simulink model "FuzzyPID_Quadrotor"  (R2025a)
settings: Solver=ode8  StartTime=0.0  StopTime=40  FixedStep=0.002  RelTol=1e-3
undefined symbols (not defined in the file): b, d, g, Ir, Ixx, Iyy, Izz, k_phi, Ki, Kp, kx, l, m
libraries: fuzblock x6, slpidlib x6, simulink x2
(part 1 of 2)
settings Model: SimulationMode=accelerator  Creator=Viết Khoa  LastModifiedBy=Viết Khoa

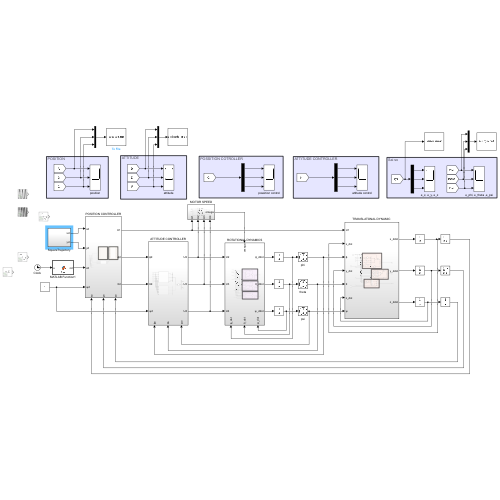
[thumbnail: Simulink's stored preview of the top-level diagram]
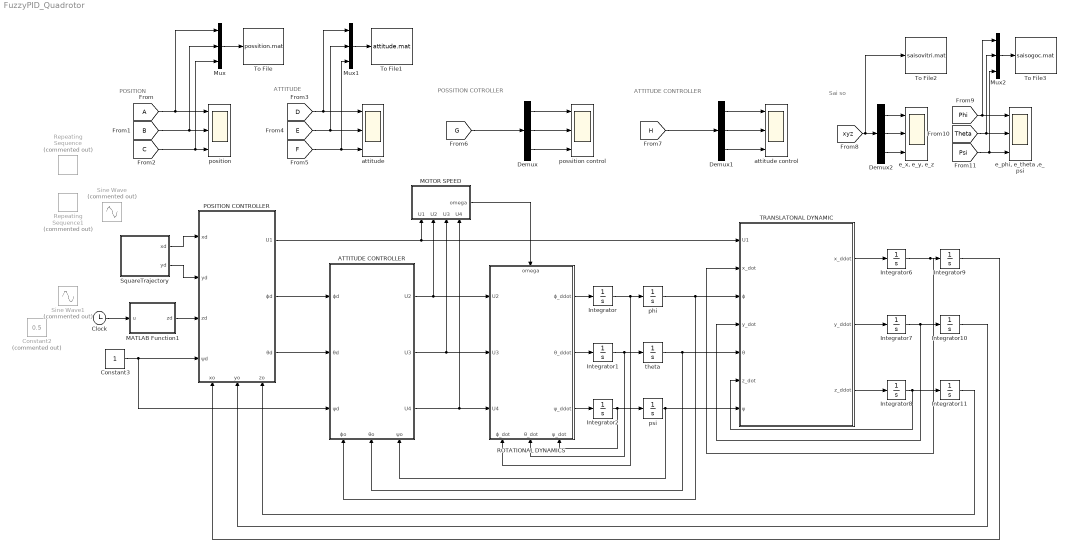
== system FuzzyPID_Quadrotor ==
  note: Sai so
  note: ATTITUDE CONTROLLER
  note: POSSITION COTROLLER
  note: ATTITUDE
  note: POSITION
  ATTITUDE CONTROLLER : Subsystem
      settings: PortSchema="{\"entries\":[{\"content\":{\"sides\":[{\"content\":{\"connectorIds\":[\"In1\",\"In2\",\"In3\"]},\"type\":\"ConnectorPlacement.EquallySpacedRectSide\",\"uuid\":\"4bf47d75-1d65-400d-a9d7-dbab3bfa16fd\"},{\"content\":{\"connectorIds\":[\"Out1\",\"Out2\",\"Out3\"],\"side\":\"RIGHT\"},\"type\":\"ConnectorPlacement.EquallySpacedRectSide\",\"uuid\":\"3ee65417-4730-4e86-9f3b-108f9b220256\"},{\"content\":{\"side\":\"TOP\"},\"type\":\"ConnectorPlacement.EquallySpacedRectSide\",\"uuid\":\"7506844b-c41f-4bd0-8d08-56ad7b5c83a6\"},{\"content\":{\"connectorIds\":[\"In4\",\"In5\",\"In6\"],\"side\":\"BOTTOM\"},\"type\":\"ConnectorPlacement.EquallySpacedRectSide\",\"uuid\":\"6a86c302-75aa-4327-998b-e6dc54af4631\"}]},\"type\":\"ConnectorPlacement.EquallySpacedConnector\",\"uuid\":\"8a896813-9530-416f-9d14-fc8134ed92a5\"}],\"packageUris\":[\"http://schema.mathworks.com/mf0/Connector/R2020b\"],\"version\":\"1.0\"}"
  Clock : Clock
      settings: Decimation=5
  Constant2 : Constant  Commented=on  Value=0.5
  Constant3 : Constant
  Demux : Demux  Outputs=3
  Demux1 : Demux  Outputs=3
  Demux2 : Demux  Outputs=3
  From : From  TagVisibility=global
  Integrator{,1..2,6..8,11} (7 alike) : Integrator
  Integrator10 : Integrator  LimitOutput=on  UpperSaturationLimit=100  LowerSaturationLimit=-100
  Integrator9 : Integrator  LimitOutput=on  UpperSaturationLimit=100  LowerSaturationLimit=-100
  MATLAB Function1 : MATLAB Function  TreatAsAtomicUnit=on
  MOTOR SPEED : Subsystem
      settings: PortSchema="{\"entries\":[{\"content\":{\"sides\":[{\"content\":{},\"type\":\"ConnectorPlacement.EquallySpacedRectSide\",\"uuid\":\"ed6e6d8d-e7bc-483a-ade7-47978a21bcb7\"},{\"content\":{\"connectorIds\":[\"Out1\"],\"side\":\"RIGHT\"},\"type\":\"ConnectorPlacement.EquallySpacedRectSide\",\"uuid\":\"acdfb20e-7f8e-459d-9194-6fd83a2c6b9b\"},{\"content\":{\"side\":\"TOP\"},\"type\":\"ConnectorPlacement.EquallySpacedRectSide\",\"uuid\":\"108cd3b7-cbe9-442f-8db2-72975fa6e768\"},{\"content\":{\"connectorIds\":[\"In1\",\"In2\",\"In3\",\"In4\"],\"side\":\"BOTTOM\"},\"type\":\"ConnectorPlacement.EquallySpacedRectSide\",\"uuid\":\"f7e31c23-3afe-47be-8aad-c67f1ef0a18a\"}]},\"type\":\"ConnectorPlacement.EquallySpacedConnector\",\"uuid\":\"b50d042a-fda9-4edf-aa4f-f774072a8c4f\"}],\"packageUris\":[\"http://schema.mathworks.com/mf0/Connector/R2020b\"],\"version\":\"1.0\"}"
  Mux : Mux  Inputs=3
  Mux1 : Mux  Inputs=3
  Mux2 : Mux  Inputs=3
  POSITION CONTROLLER : Subsystem
      settings: PortSchema="{\"entries\":[{\"content\":{\"sides\":[{\"content\":{\"connectorIds\":[\"In1\",\"In2\",\"In3\",\"In4\"]},\"type\":\"ConnectorPlacement.EquallySpacedRectSide\",\"uuid\":\"eaff3012-b374-4ff4-8d4a-29bbaff74213\"},{\"content\":{\"connectorIds\":[\"Out1\",\"Out2\",\"Out3\"],\"side\":\"RIGHT\"},\"type\":\"ConnectorPlacement.EquallySpacedRectSide\",\"uuid\":\"8b751115-4641-4ab1-9b2f-89aa7d40407f\"},{\"content\":{\"side\":\"TOP\"},\"type\":\"ConnectorPlacement.EquallySpacedRectSide\",\"uuid\":\"251f519b-9a79-4722-afff-0c5686202dfb\"},{\"content\":{\"connectorIds\":[\"In5\",\"In6\",\"In7\"],\"side\":\"BOTTOM\"},\"type\":\"ConnectorPlacement.EquallySpacedRectSide\",\"uuid\":\"18ce31f3-7bc4-45f8-83b4-9be4d1bc6b59\"}]},\"type\":\"ConnectorPlacement.EquallySpacedConnector\",\"uuid\":\"739509a0-8fec-462a-89d1-8b6a9a4571ac\"}],\"packageUris\":[\"http://schema.mathworks.com/mf0/Connector/R2020b\"],\"version\":\"1.0\"}"
  ROTATIONAL DYNAMICS : Subsystem
      settings: PortSchema="{\"entries\":[{\"content\":{\"sides\":[{\"content\":{\"connectorIds\":[\"In1\",\"In2\",\"In3\"]},\"type\":\"ConnectorPlacement.EquallySpacedRectSide\",\"uuid\":\"7bcebf77-1756-4e12-96a0-14289ff92643\"},{\"content\":{\"connectorIds\":[\"Out1\",\"Out2\",\"Out3\"],\"side\":\"RIGHT\"},\"type\":\"ConnectorPlacement.EquallySpacedRectSide\",\"uuid\":\"ba5ef720-59d3-4ec6-96cc-ef21a82cc408\"},{\"content\":{\"connectorIds\":[\"In4\"],\"side\":\"TOP\"},\"type\":\"ConnectorPlacement.EquallySpacedRectSide\",\"uuid\":\"de80adae-98be-49c2-8fe3-5182cf710150\"},{\"content\":{\"connectorIds\":[\"In5\",\"In6\",\"In7\"],\"side\":\"BOTTOM\"},\"type\":\"ConnectorPlacement.EquallySpacedRectSide\",\"uuid\":\"f6125003-ce59-4f76-bda5-387ee1b71a2b\"}]},\"type\":\"ConnectorPlacement.EquallySpacedConnector\",\"uuid\":\"a024e3ba-32fb-4ba4-b454-db7adc7fb913\"}],\"packageUris\":[\"http://schema.mathworks.com/mf0/Connector/R2020b\"],\"version\":\"1.0\"}"
  Repeating Sequence : simulink/Sources/Repeating Sequence  Commented=on  rep_seq_t=[0 2 4 6 8 10]  rep_seq_y=[0 0 2 2 0 0 ]
  Repeating Sequence1 : simulink/Sources/Repeating Sequence  Commented=on  rep_seq_t=[0 2 4 6 8 10]  rep_seq_y=[0 2 2 0 0 2 ]
  Sine Wave : Sin  Commented=on  Amplitude=2  Frequency=pi/10  SampleTime=0
  Sine Wave1 : Sin  Commented=on  Amplitude=2  Frequency=pi/10  Phase=pi/2  SampleTime=0
  SquareTrajectory : Subsystem
  "TRANSLATONAL DYNAMIC " : Subsystem
  To File : ToFile  Filename=possition.mat
  To File1 : ToFile  Filename=attitude.mat  SaveFormat=Timeseries
  To File2 : ToFile  Filename=saisovitri.mat
  To File3 : ToFile  Filename=saisogoc.mat
  attitude : Scope  NumInputPorts=3
      settings: ActiveDisplayYMinimum=-0.31829898344644053  ActiveDisplayYMaximum=0.3123395018117221
  attitude control : Scope  NumInputPorts=3
      settings: ActiveDisplayString=3  ActiveDisplayYMinimum=-26.113832641242233  ActiveDisplayYMaximum=59.012648071249139  DataLoggingVariableName=ScopeData3
  "e_phi, e_theta ,e_psi" : Scope  NumInputPorts=3
      settings: ActiveDisplayString=3  ActiveDisplayYMinimum=-0.23701033608813543  ActiveDisplayYMaximum=1.1374455928986817  YLabel=epsi  DataLoggingVariableName=ScopeData5
  "e_x, e_y, e_z" : Scope  NumInputPorts=3
      settings: ActiveDisplayString=3  ActiveDisplayYMinimum=-1.3848015109481584  ActiveDisplayYMaximum=6.8205335012164623  YLabel=ez  DataLoggingVariableName=ScopeData4
  phi : Integrator  WrapState=on
  position : Scope  NumInputPorts=3
      settings: ActiveDisplayYMinimum=-1.3944694562558515  ActiveDisplayYMaximum=12.140863842930267
  possition control : Scope  NumInputPorts=3
      settings: ActiveDisplayString=3  ActiveDisplayYMinimum=-3.1076811932529651  ActiveDisplayYMaximum=19.789742354805885  YLabel=Uz  DataLoggingVariableName=ScopeData2
  psi : Integrator  WrapState=on
  theta : Integrator  WrapState=on
  wires:
  Constant3/1 -> ATTITUDE CONTROLLER/3(ψd), POSITION CONTROLLER/4(ψd)
  POSITION CONTROLLER/2(ϕd) -> ATTITUDE CONTROLLER/1(ϕd)
  POSITION CONTROLLER/3(θd) -> ATTITUDE CONTROLLER/2(θd)
  ATTITUDE CONTROLLER/3(U4) -> ROTATIONAL DYNAMICS/3(U4), MOTOR SPEED/4(U4)
  ATTITUDE CONTROLLER/2(U3) -> MOTOR SPEED/3(U3), ROTATIONAL DYNAMICS/2(U3)
  ATTITUDE CONTROLLER/1(U2) -> ROTATIONAL DYNAMICS/1(U2), MOTOR SPEED/2(U2)
  MOTOR SPEED/1(omega) -> ROTATIONAL DYNAMICS/4(omega)
  ROTATIONAL DYNAMICS/1(ϕ_ddot) -> Integrator/1
  Integrator/1 -> ROTATIONAL DYNAMICS/5(ϕ_dot), phi/1
  ROTATIONAL DYNAMICS/2(θ_ddot) -> Integrator1/1
  Integrator1/1 -> ROTATIONAL DYNAMICS/6(θ_dot), theta/1
  ROTATIONAL DYNAMICS/3(ψ_ddot) -> Integrator2/1
  phi/1 -> ATTITUDE CONTROLLER/4(ϕo), "TRANSLATONAL DYNAMIC "/3(ϕ)
  theta/1 -> "TRANSLATONAL DYNAMIC "/5(θ), ATTITUDE CONTROLLER/5(θo)
  psi/1 -> ATTITUDE CONTROLLER/6(ψo), "TRANSLATONAL DYNAMIC "/7(ψ)
  Integrator2/1 -> ROTATIONAL DYNAMICS/7(ψ_dot), psi/1
  POSITION CONTROLLER/1(U1) -> MOTOR SPEED/1(U1), "TRANSLATONAL DYNAMIC "/1(U1)
  "TRANSLATONAL DYNAMIC "/1(x_ddot) -> Integrator6/1
  Integrator6/1 -> "TRANSLATONAL DYNAMIC "/2(x_dot), Integrator9/1
  "TRANSLATONAL DYNAMIC "/2(y_ddot) -> Integrator7/1
  Integrator7/1 -> "TRANSLATONAL DYNAMIC "/4(y_dot), Integrator10/1
  "TRANSLATONAL DYNAMIC "/3(z_ddot) -> Integrator8/1
  Integrator8/1 -> Integrator11/1, "TRANSLATONAL DYNAMIC "/6(z_dot)
  Integrator9/1 -> POSITION CONTROLLER/5(xo)
  Integrator10/1 -> POSITION CONTROLLER/6(yo)
  Integrator11/1 -> POSITION CONTROLLER/7(zo)
  [C] -> Mux/3, position/3
  [B] -> Mux/2, position/2
  From/1 -> Mux/1, position/1
  [D] -> Mux1/1, attitude/1
  [F] -> Mux1/3, attitude/3
  [E] -> Mux1/2, attitude/2
  [G] -> Demux/1
  Demux/1 -> possition control/1
  Demux/2 -> possition control/2
  Demux/3 -> possition control/3
  Demux1/3 -> attitude control/3
  Demux1/2 -> attitude control/2
  Demux1/1 -> attitude control/1
  [H] -> Demux1/1
  [Phi] -> Mux2/1, "e_phi, e_theta ,e_psi"/1
  [Theta] -> Mux2/2, "e_phi, e_theta ,e_psi"/2
  [Psi] -> Mux2/3, "e_phi, e_theta ,e_psi"/3
  [xyz] -> To File2/1, Demux2/1
  Demux2/1 -> "e_x, e_y, e_z"/1
  Demux2/2 -> "e_x, e_y, e_z"/2
  Demux2/3 -> "e_x, e_y, e_z"/3
  Clock/1 -> MATLAB Function1/1(u)
  MATLAB Function1/1(zd) -> POSITION CONTROLLER/3(zd)
  SquareTrajectory/1(xd) -> POSITION CONTROLLER/1(xd)
  SquareTrajectory/2(yd) -> POSITION CONTROLLER/2(yd)
  Mux/1 -> To File/1
  Mux1/1 -> To File1/1
  Mux2/1 -> To File3/1

== system FuzzyPID_Quadrotor/ATTITUDE CONTROLLER ==
  ϕd : Inport
  θd : Inport  Port=2
  ψd : Inport  Port=3
  ϕo : Inport  Port=4
  θo : Inport  Port=5
  ψo : Inport  Port=6
  Demux : Demux  Outputs=3
  FuzzyPID_Attitude : Subsystem
  Manual Switch : ManualSwitch
  Mux : Mux  Inputs=3
  Mux1 : Mux  Commented=on  Inputs=3
  Subsystem : Subsystem  Commented=on
  U2 : Outport
  U3 : Outport  Port=2
  U4 : Outport  Port=3
  wires:
  ϕd/1 -> Subsystem/1(ϕd), FuzzyPID_Attitude/1(ϕd)
  ϕo/1 -> Subsystem/2(ϕo), FuzzyPID_Attitude/2(ϕo)
  θd/1 -> Subsystem/3(θd), FuzzyPID_Attitude/3(θd)
  θo/1 -> Subsystem/4(θo), FuzzyPID_Attitude/4(θo)
  ψd/1 -> Subsystem/5(ψd), FuzzyPID_Attitude/5(ψd)
  ψo/1 -> Subsystem/6(ψo), FuzzyPID_Attitude/6(ψo)
  FuzzyPID_Attitude/2(U3) -> Mux/2
  FuzzyPID_Attitude/1(U2) -> Mux/1
  FuzzyPID_Attitude/3(U4) -> Mux/3
  Subsystem/2(U3) -> Mux1/2
  Subsystem/1(U2) -> Mux1/1
  Subsystem/3(U4) -> Mux1/3
  Mux/1 -> Manual Switch/1
  Mux1/1 -> Manual Switch/2
  Manual Switch/1 -> Demux/1
  Demux/3 -> U4/1
  Demux/2 -> U3/1
  Demux/1 -> U2/1

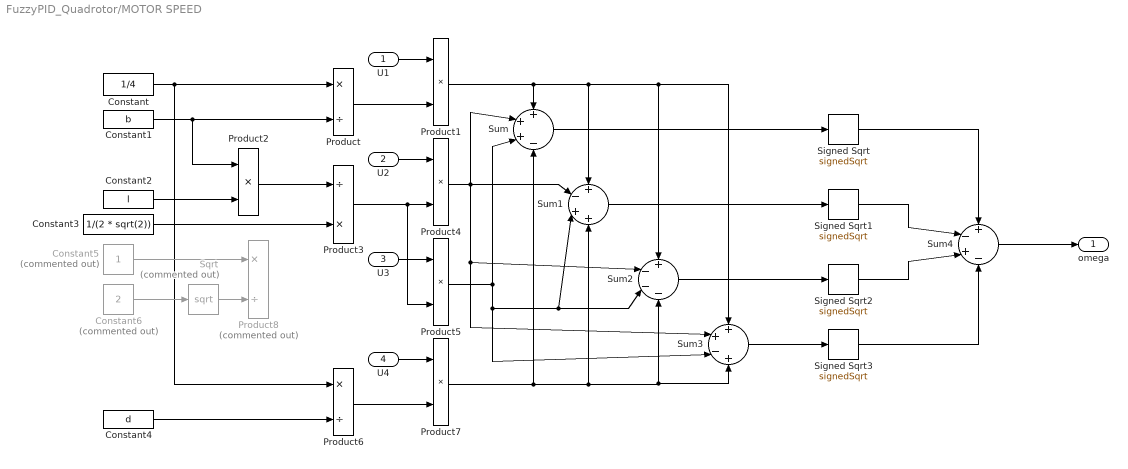
== system FuzzyPID_Quadrotor/MOTOR SPEED ==
  U1 : Inport
  U2 : Inport  Port=2
  U3 : Inport  Port=3
  U4 : Inport  Port=4
  Constant : Constant  Value=1/4
  Constant1 : Constant  Value=b
  Constant2 : Constant  Value=l
  Constant3 : Constant  Value=1/(2 * sqrt(2))
  Constant4 : Constant  Value=d
  Constant5 : Constant  Commented=on
  Constant6 : Constant  Commented=on  Value=2
  Product : Product  Inputs=*/
  Product{1..2,4..5,7} (5 alike) : Product
  Product3 : Product  Inputs=/*
  Product6 : Product  Inputs=*/
  Product8 : Product  Commented=on  Inputs=*/
  Signed Sqrt{,1..3} (4 alike) : Sqrt  Operator=signedSqrt
  Sqrt : Sqrt  Commented=on
  Sum : Sum  Inputs=+++-
  Sum1 : Sum  Inputs=+-++
  Sum2 : Sum  Inputs=+---
  Sum3 : Sum  Inputs=++-+
  Sum4 : Sum  Inputs=+-+-
  omega : Outport
  wires:
  Constant/1 -> Product6/1, Product/1
  Constant1/1 -> Product2/1, Product/2
  U1/1 -> Product1/1
  Product/1 -> Product1/2
  Constant2/1 -> Product2/2
  Product2/1 -> Product3/1
  U2/1 -> Product4/1
  Product3/1 -> Product5/2, Product4/2
  U3/1 -> Product5/1
  Constant4/1 -> Product6/2
  Product6/1 -> Product7/2
  U4/1 -> Product7/1
  Product1/1 -> Sum/1, Sum2/1, Sum3/1, Sum1/1
  Product4/1 -> Sum2/2, Sum3/2, Sum/2, Sum1/2
  Product5/1 -> Sum3/3, Sum1/3, Sum2/3, Sum/3
  Product7/1 -> Sum/4, Sum3/4, Sum2/4, Sum1/4
  Sum/1 -> Signed Sqrt/1
  Sum1/1 -> Signed Sqrt1/1
  Sum2/1 -> Signed Sqrt2/1
  Sum3/1 -> Signed Sqrt3/1
  Signed Sqrt/1 -> Sum4/1
  Signed Sqrt1/1 -> Sum4/2
  Signed Sqrt2/1 -> Sum4/3
  Signed Sqrt3/1 -> Sum4/4
  Sum4/1 -> omega/1
  Constant6/1 -> Sqrt/1
  Sqrt/1 -> Product8/2
  Constant5/1 -> Product8/1
  Constant3/1 -> Product3/2

== system FuzzyPID_Quadrotor/POSITION CONTROLLER ==
  note: CACULATION DESIRED ROLL AND PITCH, THUST
  note: BỘ ĐIỀU KHIỂN VỊ TRÍ
  xd : Inport
  yd : Inport  Port=2
  zd : Inport  Port=3
  ψd : Inport  Port=4
  xo : Inport  Port=5
  yo : Inport  Port=6
  zo : Inport  Port=7
  Demux : Demux  Commented=on  Outputs=6
  Demux1 : Demux  Outputs=6
  FUZZY PID POSITION : Subsystem  Commented=on
  Goto : Goto  TagVisibility=global
  Mux : Mux  Inputs=6
  Mux1 : Mux  Inputs=2
  Mux2 : Mux  Inputs=2
  Mux3 : Mux  Inputs=2
  Subsystem : Subsystem
      settings: PortSchema="{\"entries\":[{\"content\":{\"sides\":[{\"content\":{\"connectorIds\":[\"In1\",\"In2\",\"In3\"]},\"type\":\"ConnectorPlacement.EquallySpacedRectSide\",\"uuid\":\"734b09d6-8ba9-424b-aad8-7b68aeaa8799\"},{\"content\":{\"connectorIds\":[\"Out1\",\"Out2\",\"Out3\"],\"side\":\"RIGHT\"},\"type\":\"ConnectorPlacement.EquallySpacedRectSide\",\"uuid\":\"ae7a8814-eaf7-43aa-9eb5-210d717eae53\"},{\"content\":{\"side\":\"TOP\"},\"type\":\"ConnectorPlacement.EquallySpacedRectSide\",\"uuid\":\"c79c257a-0698-4fb1-979a-f95adc922051\"},{\"content\":{\"connectorIds\":[\"In4\"],\"side\":\"BOTTOM\"},\"type\":\"ConnectorPlacement.EquallySpacedRectSide\",\"uuid\":\"97cb2459-45e5-4eb8-bf6c-59a8c59ceda8\"}]},\"type\":\"ConnectorPlacement.EquallySpacedConnector\",\"uuid\":\"b23e5638-8d2f-4e41-ba88-ebe95de464d7\"}],\"packageUris\":[\"http://schema.mathworks.com/mf0/Connector/R2020b\"],\"version\":\"1.0\"}"
  Subsystem2 : Subsystem
  U1 : Outport
  ϕd : Outport  Port=2
  θd : Outport  Port=3
  tag scope: B=global, C=global
  wires:
  ψd/1 -> Subsystem/4(ψd)
  Subsystem/1(U1) -> U1/1
  Subsystem/2(ϕd) -> ϕd/1
  Subsystem/3(θd) -> θd/1
  xd/1 -> Mux/1, Mux1/1
  yd/1 -> Mux2/1, Mux/2
  zd/1 -> Mux3/1, Mux/3
  xo/1 -> Mux/4, Mux1/2
  yo/1 -> Mux2/2, Mux/5
  zo/1 -> Mux3/2, Mux/6
  Demux/6 -> FUZZY PID POSITION/6(zo)
  Demux/5 -> FUZZY PID POSITION/5(yo)
  Demux/4 -> FUZZY PID POSITION/4(xo)
  Demux/3 -> FUZZY PID POSITION/3(zd)
  Demux/2 -> FUZZY PID POSITION/2(yd)
  Demux/1 -> FUZZY PID POSITION/1(xd)
  Mux/1 -> Demux/1, Demux1/1
  Demux1/1 -> Subsystem2/1(xd)
  Demux1/2 -> Subsystem2/2(yd)
  Demux1/3 -> Subsystem2/3(zd)
  Demux1/4 -> Subsystem2/4(xo)
  Demux1/5 -> Subsystem2/5(yo)
  Demux1/6 -> Subsystem2/6(zo)
  Mux1/1 -> Goto/1
  Mux2/1 -> [B]
  Mux3/1 -> [C]
  Subsystem2/1(Ux) -> Subsystem/1(Ux)
  Subsystem2/2(Uy) -> Subsystem/2(Uy)
  Subsystem2/3(Uz) -> Subsystem/3(Uz)

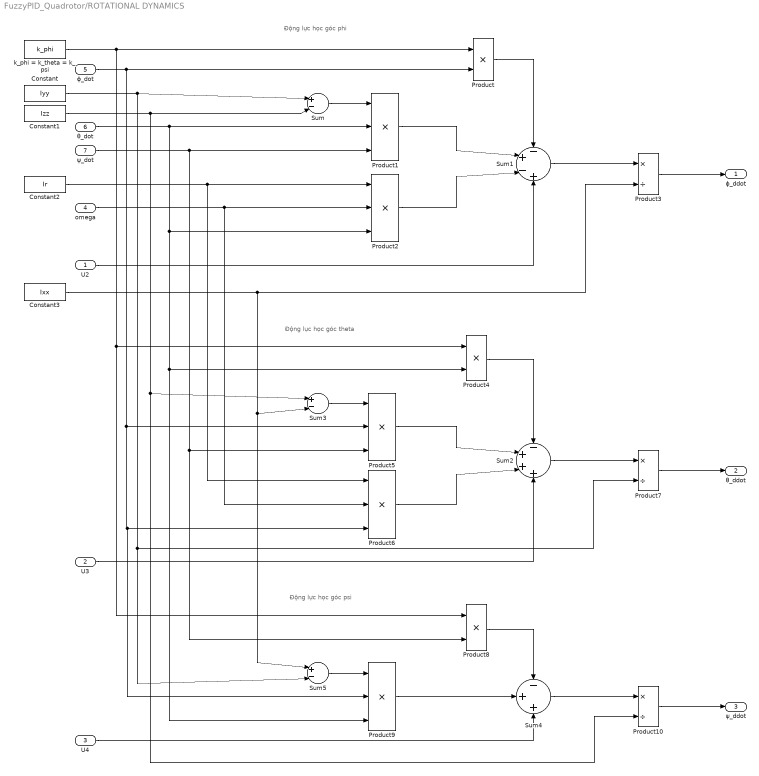
== system FuzzyPID_Quadrotor/ROTATIONAL DYNAMICS ==
  note: Động lực học góc psi
  note: Động lục học góc theta
  note: Động lực học góc phi
  U2 : Inport
  U3 : Inport  Port=2
  U4 : Inport  Port=3
  omega : Inport  Port=4
  ϕ_dot : Inport  Port=5
  θ_dot : Inport  Port=6
  ψ_dot : Inport  Port=7
  Constant : Constant  Value=Iyy
  Constant1 : Constant  Value=Izz
  Constant2 : Constant  Value=Ir
  Constant3 : Constant  Value=Ixx
  Product : Product
  Product{1..2,5..6,9} (5 alike) : Product  Inputs=3
  Product10 : Product  Inputs=*/
  Product3 : Product  Inputs=*/
  Product4 : Product
  Product7 : Product  Inputs=*/
  Product8 : Product
  Sum : Sum  Inputs=|+-|
  Sum1 : Sum  Inputs=-+-+
  Sum2 : Sum  Inputs=-+++
  Sum3 : Sum  Inputs=|+-|
  Sum4 : Sum  Inputs=-++
  Sum5 : Sum  Inputs=|+-|
  k_phi = k_theta = k_psi : Constant  Value=k_phi
  ϕ_ddot : Outport
  θ_ddot : Outport  Port=2
  ψ_ddot : Outport  Port=3
  wires:
  k_phi = k_theta = k_psi/1 -> Product8/1, Product4/1, Product/1
  ϕ_dot/1 -> Product/2, Product5/2, Product9/2, Product6/3
  Constant/1 -> Product7/2, Sum5/2, Sum/1
  Constant1/1 -> Sum3/1, Product10/2, Sum/2
  Sum/1 -> Product1/1
  Product/1 -> Sum1/1
  Product1/1 -> Sum1/2
  Constant2/1 -> Product6/1, Product2/1
  omega/1 -> Product6/2, Product2/2
  Product2/1 -> Sum1/3
  U2/1 -> Sum1/4
  Sum1/1 -> Product3/1
  Constant3/1 -> Sum3/2, Sum5/1, Product3/2
  Product3/1 -> ϕ_ddot/1
  θ_dot/1 -> Product4/2, Product9/3, Product2/3, Product1/2
  Product4/1 -> Sum2/1
  Sum3/1 -> Product5/1
  Product5/1 -> Sum2/2
  Product6/1 -> Sum2/3
  Sum2/1 -> Product7/1
  Product7/1 -> θ_ddot/1
  ψ_dot/1 -> Product8/2, Product5/3, Product1/3
  Product8/1 -> Sum4/1
  Sum5/1 -> Product9/1
  Product9/1 -> Sum4/2
  U3/1 -> Sum2/4
  U4/1 -> Sum4/3
  Sum4/1 -> Product10/1
  Product10/1 -> ψ_ddot/1

== system FuzzyPID_Quadrotor/SquareTrajectory ==
  Clock : Clock
      settings: Decimation=5
  Clock1 : Clock
      settings: Decimation=5
  MATLAB Function : MATLAB Function  TreatAsAtomicUnit=on
  MATLAB Function1 : MATLAB Function  TreatAsAtomicUnit=on
  To Workspace : ToWorkspace  VariableName=Time  SampleTime=-1
  To Workspace1 : ToWorkspace  VariableName=xd  SampleTime=-1
  To Workspace2 : ToWorkspace  VariableName=yd  SampleTime=-1
  xd : Outport
  yd : Outport  Port=2
  wires:
  Clock/1 -> MATLAB Function1/1(u), MATLAB Function/1(u)
  Clock1/1 -> To Workspace/1
  MATLAB Function1/1(xd) -> To Workspace1/1, xd/1
  MATLAB Function/1(yd) -> To Workspace2/1, yd/1

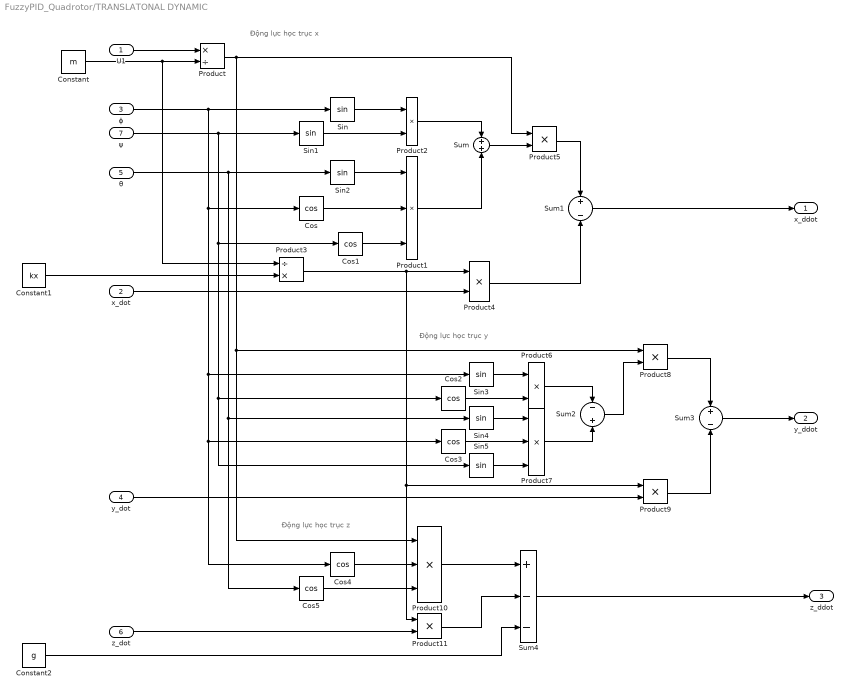
== system FuzzyPID_Quadrotor/TRANSLATONAL DYNAMIC  ==
  note: Động lực học trục z
  note: Động lực học trục y
  note: Động lực học trục x
  U1 : Inport
  x_dot : Inport  Port=2
  ϕ : Inport  Port=3
  y_dot : Inport  Port=4
  θ : Inport  Port=5
  z_dot : Inport  Port=6
  ψ : Inport  Port=7
  Constant : Constant  Value=m
  Constant1 : Constant  Value=kx
  Constant2 : Constant  Value=g
  Cos{,1..5} (6 alike) : Trigonometry  Operator=cos
  Product : Product  Inputs=*/
  Product1 : Product  Inputs=3
  Product10 : Product  Inputs=3
  Product{2,4..6,8..9,11} (7 alike) : Product
  Product3 : Product  Inputs=/*
  Product7 : Product  Inputs=3
  Sin{,1..5} (6 alike) : Trigonometry
  Sum : Sum  Inputs=+|+
  Sum1 : Sum  Inputs=+|-
  Sum2 : Sum  Inputs=-|+
  Sum3 : Sum  Inputs=+|-
  Sum4 : Sum  Inputs=+--
  x_ddot : Outport
  y_ddot : Outport  Port=2
  z_ddot : Outport  Port=3
  wires:
  U1/1 -> Product/1
  Constant/1 -> Product/2, Product3/1
  ϕ/1 -> Sin/1, Cos/1, Sin3/1, Cos4/1, Cos3/1
  Sin/1 -> Product2/1
  ψ/1 -> Sin1/1, Cos1/1, Cos2/1, Sin5/1
  Sin1/1 -> Product2/2
  θ/1 -> Sin4/1, Cos5/1, Sin2/1
  Sin2/1 -> Product1/1
  Cos/1 -> Product1/2
  Cos1/1 -> Product1/3
  Product2/1 -> Sum/1
  Product1/1 -> Sum/2
  Constant1/1 -> Product3/2
  Product3/1 -> Product11/1, Product9/1, Product4/1
  x_dot/1 -> Product4/2
  Product4/1 -> Sum1/2
  Sum/1 -> Product5/2
  Product5/1 -> Sum1/1
  Sin3/1 -> Product6/1
  Cos2/1 -> Product6/2
  Sin4/1 -> Product7/1
  Cos3/1 -> Product7/2
  Sin5/1 -> Product7/3
  Product6/1 -> Sum2/1
  Product7/1 -> Sum2/2
  Sum2/1 -> Product8/2
  y_dot/1 -> Product9/2
  Product8/1 -> Sum3/1
  Product9/1 -> Sum3/2
  Product/1 -> Product8/1, Product10/1, Product5/1
  Cos4/1 -> Product10/2
  Cos5/1 -> Product10/3
  z_dot/1 -> Product11/2
  Product10/1 -> Sum4/1
  Product11/1 -> Sum4/2
  Constant2/1 -> Sum4/3
  Sum1/1 -> x_ddot/1
  Sum3/1 -> y_ddot/1
  Sum4/1 -> z_ddot/1

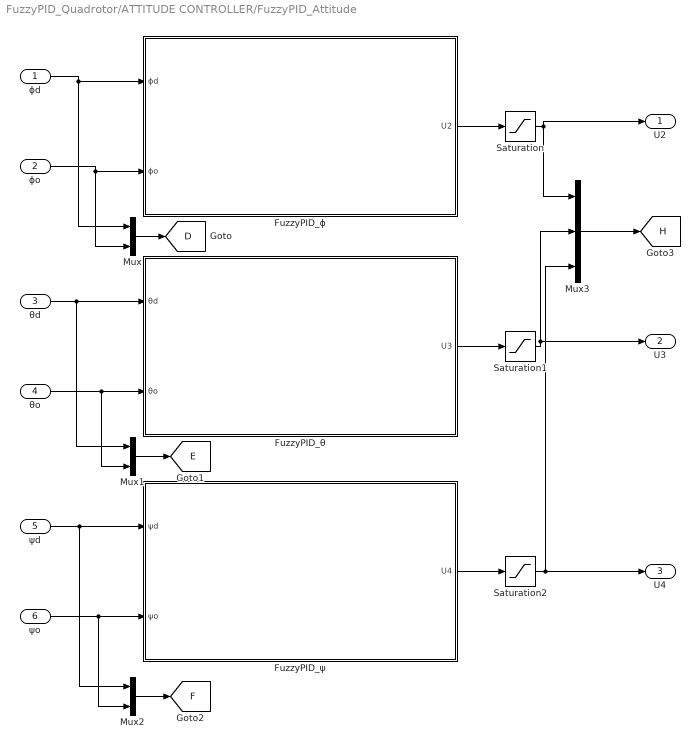
== system FuzzyPID_Quadrotor/ATTITUDE CONTROLLER/FuzzyPID_Attitude ==
  ϕd : Inport
  ϕo : Inport  Port=2
  θd : Inport  Port=3
  θo : Inport  Port=4
  ψd : Inport  Port=5
  ψo : Inport  Port=6
  FuzzyPID_θ : Subsystem
  FuzzyPID_ψ : Subsystem
  FuzzyPID_ϕ : Subsystem
  Mux : Mux  Inputs=2
  Mux1 : Mux  Inputs=2
  Mux2 : Mux  Inputs=2
  Mux3 : Mux  Inputs=3
  Saturation : Saturate  UpperLimit=500  LowerLimit=-500
  Saturation1 : Saturate  UpperLimit=500  LowerLimit=-500
  Saturation2 : Saturate  UpperLimit=500  LowerLimit=-500
  U2 : Outport
  U3 : Outport  Port=2
  U4 : Outport  Port=3
  tag scope: D=global, E=global, F=global, H=global
  wires:
  ϕd/1 -> Mux/1, FuzzyPID_ϕ/1(ϕd)
  ψd/1 -> Mux2/1, FuzzyPID_ψ/1(ψd)
  Saturation1/1 -> U3/1, Mux3/2
  ψo/1 -> Mux2/2, FuzzyPID_ψ/2(ψo)
  Mux2/1 -> [F]
  ϕo/1 -> Mux/2, FuzzyPID_ϕ/2(ϕo)
  Saturation/1 -> U2/1, Mux3/1
  θo/1 -> Mux1/2, FuzzyPID_θ/2(θo)
  FuzzyPID_ψ/1(U4) -> Saturation2/1
  Saturation2/1 -> U4/1, Mux3/3
  Mux/1 -> [D]
  θd/1 -> Mux1/1, FuzzyPID_θ/1(θd)
  FuzzyPID_ϕ/1(U2) -> Saturation/1
  FuzzyPID_θ/1(U3) -> Saturation1/1
  Mux3/1 -> [H]
  Mux1/1 -> [E]

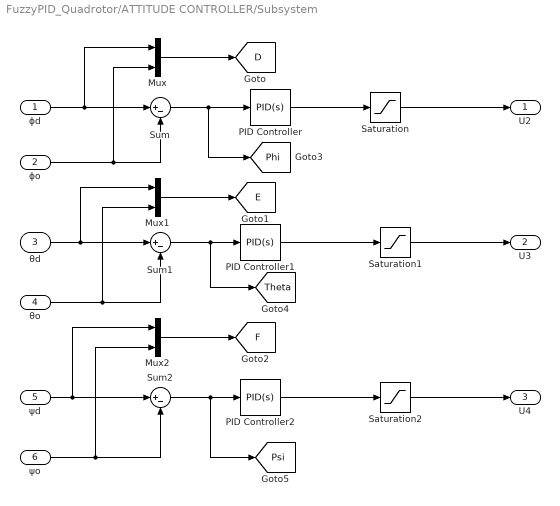
== system FuzzyPID_Quadrotor/ATTITUDE CONTROLLER/Subsystem ==
  ϕd : Inport
  ϕo : Inport  Port=2
  θd : Inport  Port=3
  θo : Inport  Port=4
  ψd : Inport  Port=5
  ψo : Inport  Port=6
  Mux : Mux  Inputs=2
  Mux1 : Mux  Inputs=2
  Mux2 : Mux  Inputs=2
  PID Controller : slpidlib/PID Controller  Controller=PID  Form=Parallel  TimeDomain=Continuous-time  UseExternalTs=off  SampleTime=-1  IntegratorMethod=Forward Euler  FilterMethod=Forward Euler  ControllerParametersSource=internal  P=1  I=0.01  UseKiTs=off  D=0.1  UseExternalDerivativeSource=off  N=0.0166910746973265  UseFilter=on  TunerSelectOption=Transfer Function Based (PID Tuner App)  InitialConditionSource=internal  InitialConditionForIntegrator=0  InitialConditionForFilter=0  DifferentiatorICPrevScaledInput=0  ExternalReset=none  TrackingMode=off  Kt=1  LimitOutput=off  SatLimitsSource=internal  UpperSaturationLimit=inf  LowerSaturationLimit=-inf  LinearizeAsGain=on  AntiWindupMode=none  Kb=1  LimitIntegrator=off  UpperIntegratorSaturationLimit=inf  LowerIntegratorSaturationLimit=-inf  POutMin=[]  POutMax=[]  IOutMin=[]  IOutMax=[]  DOutMin=[]  DOutMax=[]  NOutMin=[]  NOutMax=[]  SumOutMin=[]  SumOutMax=[]  SaturationOutMin=[]  SaturationOutMax=[]  PParamMin=[]  PParamMax=[]  IParamMin=[]  IParamMax=[]  DParamMin=[]  DParamMax=[]  NParamMin=[]  NParamMax=[]  KbParamMin=[]  KbParamMax=[]  KtParamMin=[]  KtParamMax=[]  KbOutMin=[]  KbOutMax=[]  KtOutMin=[]  KtOutMax=[]  IntegratorOutMin=[]  IntegratorOutMax=[]  FilterOutMin=[]  FilterOutMax=[]  SumI1OutMin=[]  SumI1OutMax=[]  SumI2OutMin=[]  SumI2OutMax=[]  SumI3OutMin=[]  SumI3OutMax=[]  SumI4OutMin=[]  SumI4OutMax=[]  SumDOutMin=[]  SumDOutMax=[]  DifferentiatorOutMin=[]  DifferentiatorOutMax=[]  FilterDiffOutCoefMin=[]  FilterDiffOutCoefMax=[]  ReciprocalOutMin=[]  ReciprocalOutMax=[]  SumDenOutMin=[]  SumDenOutMax=[]  SumNumOutMin=[]  SumNumOutMax=[]  DivideOutMin=[]  DivideOutMax=[]  UdiffTsProdOutMin=[]  UdiffTsProdOutMax=[]  NTsProdOutMin=[]  NTsProdOutMax=[]  UintegralTsProdOutMin=[]  UintegralTsProdOutMax=[]  UngainTsProdOutMin=[]  UngainTsProdOutMax=[]  ClampingZeroOutDataTypeStr=Inherit: Inherit via back propagation  ClampingZeroOutMin=[]  ClampingZeroOutMax=[]  FilterDenConstantOutDataTypeStr=Inherit: Inherit via back propagation  FilterDenConstantOutMin=[]  FilterDenConstantOutMax=[]  PCopyOutDataTypeStr=Inherit: Inherit via back propagation  PCopyOutMin=[]  PCopyOutMax=[]  NCopyOutDataTypeStr=Inherit: Inherit via back propagation  NCopyOutMin=[]  NCopyOutMax=[]  IntegratorContinuousStateAttributes=''  IntegratorStateMustResolveToSignalObject=off  IntegratorRTWStateStorageClass=Auto  FilterContinuousStateAttributes=''  FilterStateMustResolveToSignalObject=off  FilterRTWStateStorageClass=Auto  ParallelPVariant=InternalParameters  IdealPVariant=Disabled  IVariant=InternalParameters  DVariant=InternalParameters  IntegratorVariant=Continuous  SatVariant=Disabled  AWVariant=Passthrough  PCopyVariant=Disabled  TRVariant=Disabled  FdbkBlocksVariant=Forward  IdealPFdbkVariant=Disabled  SatFdbkVariant=Disabled  DerivativeFilterVariant=ContFilter  NVariant=InternalParameters  NCopyVariant=Disabled  FilterICVariant=InternalICsFilter  IntegratorICVariant=InternalICs  ExternalResetVariant=Disabled  TRSumVariant=Passthrough  SumFdbkVariant=Disabled  SumVariant=Sum_PID  TsampFilterVariant=InternalTs  TsampNgainVariant=Passthrough  TsampIntegralVariant=Disabled_SignalSpec  ExternalSaturationOutDataTypeStr=Inherit: Same as second input  DerivativeSourceVariant=ErrorSignal  PreIntVariant=InternalPreInt
  PID Controller1 : slpidlib/PID Controller  Controller=PID  Form=Parallel  TimeDomain=Continuous-time  UseExternalTs=off  SampleTime=-1  IntegratorMethod=Forward Euler  FilterMethod=Forward Euler  ControllerParametersSource=internal  P=1  I=0.01  UseKiTs=off  D=0.1  UseExternalDerivativeSource=off  N=100  UseFilter=on  TunerSelectOption=Transfer Function Based (PID Tuner App)  InitialConditionSource=internal  InitialConditionForIntegrator=0  InitialConditionForFilter=0  DifferentiatorICPrevScaledInput=0  ExternalReset=none  TrackingMode=off  Kt=1  LimitOutput=off  SatLimitsSource=internal  UpperSaturationLimit=inf  LowerSaturationLimit=-inf  LinearizeAsGain=on  AntiWindupMode=none  Kb=1  LimitIntegrator=off  UpperIntegratorSaturationLimit=inf  LowerIntegratorSaturationLimit=-inf  POutMin=[]  POutMax=[]  IOutMin=[]  IOutMax=[]  DOutMin=[]  DOutMax=[]  NOutMin=[]  NOutMax=[]  SumOutMin=[]  SumOutMax=[]  SaturationOutMin=[]  SaturationOutMax=[]  PParamMin=[]  PParamMax=[]  IParamMin=[]  IParamMax=[]  DParamMin=[]  DParamMax=[]  NParamMin=[]  NParamMax=[]  KbParamMin=[]  KbParamMax=[]  KtParamMin=[]  KtParamMax=[]  KbOutMin=[]  KbOutMax=[]  KtOutMin=[]  KtOutMax=[]  IntegratorOutMin=[]  IntegratorOutMax=[]  FilterOutMin=[]  FilterOutMax=[]  SumI1OutMin=[]  SumI1OutMax=[]  SumI2OutMin=[]  SumI2OutMax=[]  SumI3OutMin=[]  SumI3OutMax=[]  SumI4OutMin=[]  SumI4OutMax=[]  SumDOutMin=[]  SumDOutMax=[]  DifferentiatorOutMin=[]  DifferentiatorOutMax=[]  FilterDiffOutCoefMin=[]  FilterDiffOutCoefMax=[]  ReciprocalOutMin=[]  ReciprocalOutMax=[]  SumDenOutMin=[]  SumDenOutMax=[]  SumNumOutMin=[]  SumNumOutMax=[]  DivideOutMin=[]  DivideOutMax=[]  UdiffTsProdOutMin=[]  UdiffTsProdOutMax=[]  NTsProdOutMin=[]  NTsProdOutMax=[]  UintegralTsProdOutMin=[]  UintegralTsProdOutMax=[]  UngainTsProdOutMin=[]  UngainTsProdOutMax=[]  ClampingZeroOutDataTypeStr=Inherit: Inherit via back propagation  ClampingZeroOutMin=[]  ClampingZeroOutMax=[]  FilterDenConstantOutDataTypeStr=Inherit: Inherit via back propagation  FilterDenConstantOutMin=[]  FilterDenConstantOutMax=[]  PCopyOutDataTypeStr=Inherit: Inherit via back propagation  PCopyOutMin=[]  PCopyOutMax=[]  NCopyOutDataTypeStr=Inherit: Inherit via back propagation  NCopyOutMin=[]  NCopyOutMax=[]  IntegratorContinuousStateAttributes=''  IntegratorStateMustResolveToSignalObject=off  IntegratorRTWStateStorageClass=Auto  FilterContinuousStateAttributes=''  FilterStateMustResolveToSignalObject=off  FilterRTWStateStorageClass=Auto  ParallelPVariant=InternalParameters  IdealPVariant=Disabled  IVariant=InternalParameters  DVariant=InternalParameters  IntegratorVariant=Continuous  SatVariant=Disabled  AWVariant=Passthrough  PCopyVariant=Disabled  TRVariant=Disabled  FdbkBlocksVariant=Forward  IdealPFdbkVariant=Disabled  SatFdbkVariant=Disabled  DerivativeFilterVariant=ContFilter  NVariant=InternalParameters  NCopyVariant=Disabled  FilterICVariant=InternalICsFilter  IntegratorICVariant=InternalICs  ExternalResetVariant=Disabled  TRSumVariant=Passthrough  SumFdbkVariant=Disabled  SumVariant=Sum_PID  TsampFilterVariant=InternalTs  TsampNgainVariant=Passthrough  TsampIntegralVariant=Disabled_SignalSpec  ExternalSaturationOutDataTypeStr=Inherit: Same as second input  DerivativeSourceVariant=ErrorSignal  PreIntVariant=InternalPreInt
  PID Controller2 : slpidlib/PID Controller  Controller=PID  Form=Parallel  TimeDomain=Continuous-time  UseExternalTs=off  SampleTime=-1  IntegratorMethod=Forward Euler  FilterMethod=Forward Euler  ControllerParametersSource=internal  P=1  I=0.01  UseKiTs=off  D=0.1  UseExternalDerivativeSource=off  N=100  UseFilter=on  TunerSelectOption=Transfer Function Based (PID Tuner App)  InitialConditionSource=internal  InitialConditionForIntegrator=0  InitialConditionForFilter=0  DifferentiatorICPrevScaledInput=0  ExternalReset=none  TrackingMode=off  Kt=1  LimitOutput=off  SatLimitsSource=internal  UpperSaturationLimit=inf  LowerSaturationLimit=-inf  LinearizeAsGain=on  AntiWindupMode=none  Kb=1  LimitIntegrator=off  UpperIntegratorSaturationLimit=inf  LowerIntegratorSaturationLimit=-inf  POutMin=[]  POutMax=[]  IOutMin=[]  IOutMax=[]  DOutMin=[]  DOutMax=[]  NOutMin=[]  NOutMax=[]  SumOutMin=[]  SumOutMax=[]  SaturationOutMin=[]  SaturationOutMax=[]  PParamMin=[]  PParamMax=[]  IParamMin=[]  IParamMax=[]  DParamMin=[]  DParamMax=[]  NParamMin=[]  NParamMax=[]  KbParamMin=[]  KbParamMax=[]  KtParamMin=[]  KtParamMax=[]  KbOutMin=[]  KbOutMax=[]  KtOutMin=[]  KtOutMax=[]  IntegratorOutMin=[]  IntegratorOutMax=[]  FilterOutMin=[]  FilterOutMax=[]  SumI1OutMin=[]  SumI1OutMax=[]  SumI2OutMin=[]  SumI2OutMax=[]  SumI3OutMin=[]  SumI3OutMax=[]  SumI4OutMin=[]  SumI4OutMax=[]  SumDOutMin=[]  SumDOutMax=[]  DifferentiatorOutMin=[]  DifferentiatorOutMax=[]  FilterDiffOutCoefMin=[]  FilterDiffOutCoefMax=[]  ReciprocalOutMin=[]  ReciprocalOutMax=[]  SumDenOutMin=[]  SumDenOutMax=[]  SumNumOutMin=[]  SumNumOutMax=[]  DivideOutMin=[]  DivideOutMax=[]  UdiffTsProdOutMin=[]  UdiffTsProdOutMax=[]  NTsProdOutMin=[]  NTsProdOutMax=[]  UintegralTsProdOutMin=[]  UintegralTsProdOutMax=[]  UngainTsProdOutMin=[]  UngainTsProdOutMax=[]  ClampingZeroOutDataTypeStr=Inherit: Inherit via back propagation  ClampingZeroOutMin=[]  ClampingZeroOutMax=[]  FilterDenConstantOutDataTypeStr=Inherit: Inherit via back propagation  FilterDenConstantOutMin=[]  FilterDenConstantOutMax=[]  PCopyOutDataTypeStr=Inherit: Inherit via back propagation  PCopyOutMin=[]  PCopyOutMax=[]  NCopyOutDataTypeStr=Inherit: Inherit via back propagation  NCopyOutMin=[]  NCopyOutMax=[]  IntegratorContinuousStateAttributes=''  IntegratorStateMustResolveToSignalObject=off  IntegratorRTWStateStorageClass=Auto  FilterContinuousStateAttributes=''  FilterStateMustResolveToSignalObject=off  FilterRTWStateStorageClass=Auto  ParallelPVariant=InternalParameters  IdealPVariant=Disabled  IVariant=InternalParameters  DVariant=InternalParameters  IntegratorVariant=Continuous  SatVariant=Disabled  AWVariant=Passthrough  PCopyVariant=Disabled  TRVariant=Disabled  FdbkBlocksVariant=Forward  IdealPFdbkVariant=Disabled  SatFdbkVariant=Disabled  DerivativeFilterVariant=ContFilter  NVariant=InternalParameters  NCopyVariant=Disabled  FilterICVariant=InternalICsFilter  IntegratorICVariant=InternalICs  ExternalResetVariant=Disabled  TRSumVariant=Passthrough  SumFdbkVariant=Disabled  SumVariant=Sum_PID  TsampFilterVariant=InternalTs  TsampNgainVariant=Passthrough  TsampIntegralVariant=Disabled_SignalSpec  ExternalSaturationOutDataTypeStr=Inherit: Same as second input  DerivativeSourceVariant=ErrorSignal  PreIntVariant=InternalPreInt
  Saturation : Saturate  UpperLimit=500  LowerLimit=-500
  Saturation1 : Saturate  UpperLimit=500  LowerLimit=-500
  Saturation2 : Saturate  UpperLimit=500  LowerLimit=-500
  Sum : Sum  Inputs=|+-
  Sum1 : Sum  Inputs=|+-
  Sum2 : Sum  Inputs=|+-
  U2 : Outport
  U3 : Outport  Port=2
  U4 : Outport  Port=3
  tag scope: D=global, E=global, F=global, Phi=global, Psi=global, Theta=global
  wires:
  ϕd/1 -> Mux/1, Sum/1
  ϕo/1 -> Mux/2, Sum/2
  Sum/1 -> [Phi], PID Controller/1
  PID Controller/1 -> Saturation/1
  Saturation/1 -> U2/1
  θd/1 -> Mux1/1, Sum1/1
  Sum1/1 -> [Theta], PID Controller1/1
  θo/1 -> Mux1/2, Sum1/2
  PID Controller1/1 -> Saturation1/1
  Saturation1/1 -> U3/1
  Sum2/1 -> [Psi], PID Controller2/1
  ψd/1 -> Mux2/1, Sum2/1
  ψo/1 -> Mux2/2, Sum2/2
  PID Controller2/1 -> Saturation2/1
  Saturation2/1 -> U4/1
  Mux/1 -> [D]
  Mux1/1 -> [E]
  Mux2/1 -> [F]

== system FuzzyPID_Quadrotor/POSITION CONTROLLER/FUZZY PID POSITION ==
  xd : Inport
  yd : Inport  Port=2
  zd : Inport  Port=3
  xo : Inport  Port=4
  yo : Inport  Port=5
  zo : Inport  Port=6
  FuzzyPID_x : Subsystem  mask{Kp_x=pi/2, Ki_x=0, Kd_x=pi/2}
  FuzzyPID_y : Subsystem  mask{Kp_y=pi/2, Ki_y=0, Kd_y=2*pi/3}
  FuzzyPID_z : Subsystem  mask{Kp_z=35, Ki_z=6, Kd_z=28}
  Ux : Outport
  Uy : Outport  Port=2
  Uz : Outport  Port=3
  wires:
  xd/1 -> FuzzyPID_x/1(xd)
  xo/1 -> FuzzyPID_x/2(xo)
  yo/1 -> FuzzyPID_y/2(yo)
  FuzzyPID_y/1(Uy) -> Uy/1
  FuzzyPID_z/1(Uz) -> Uz/1
  zo/1 -> FuzzyPID_z/2(zo)
  zd/1 -> FuzzyPID_z/1(zd)
  yd/1 -> FuzzyPID_y/1(yd)
  FuzzyPID_x/1(Ux) -> Ux/1

== system FuzzyPID_Quadrotor/POSITION CONTROLLER/Subsystem ==
  Ux : Inport
  Uy : Inport  Port=2
  Uz : Inport  Port=3
  ψd : Inport  Port=4
  "Roll " : Subsystem
  Theta : Subsystem
  Thrust : Subsystem
  U1 : Outport
  ϕd : Outport  Port=2
  θd : Outport  Port=3
  wires:
  Ux/1 -> Theta/1(Ux), "Roll "/1(Ux), Thrust/1(Ux)
  Uy/1 -> Theta/2(Uy), "Roll "/2(Uy), Thrust/2(Uy)
  Uz/1 -> Theta/3(Uz), "Roll "/3(Uz), Thrust/3(Uz)
  Thrust/1(U1) -> U1/1
  ψd/1 -> Theta/4(ψd), "Roll "/4(ψd)
  "Roll "/1(ϕd) -> ϕd/1
  Theta/1(θd) -> θd/1

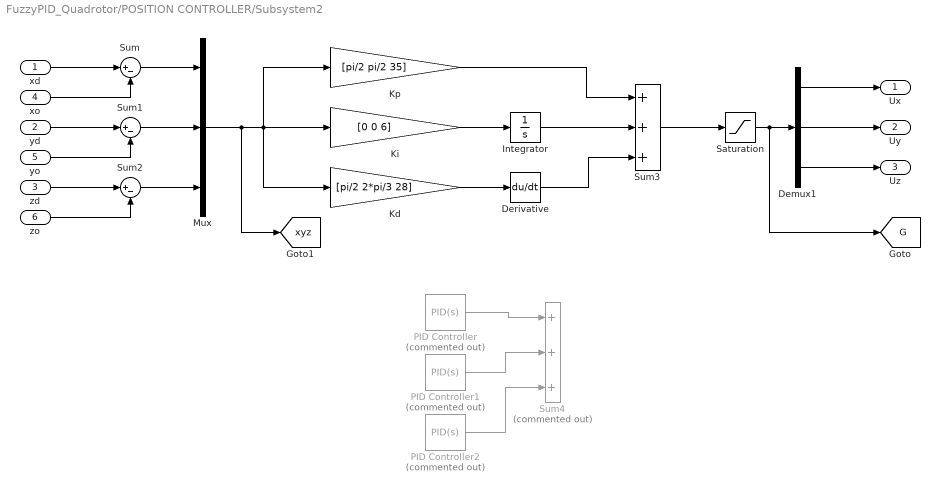
== system FuzzyPID_Quadrotor/POSITION CONTROLLER/Subsystem2 ==
  xd : Inport
  yd : Inport  Port=2
  zd : Inport  Port=3
  xo : Inport  Port=4
  yo : Inport  Port=5
  zo : Inport  Port=6
  Demux1 : Demux  Outputs=3
  Derivative : Derivative
  Integrator : Integrator
  Kd : Gain  Gain=[pi/2 2*pi/3 28]
  Ki : Gain  Gain=[0 0 6]
  Kp : Gain  Gain=[pi/2 pi/2 35]
  Mux : Mux  Inputs=3
  PID Controller : slpidlib/PID Controller  Commented=on  Controller=PID  Form=Parallel  TimeDomain=Continuous-time  UseExternalTs=off  SampleTime=-1  IntegratorMethod=Forward Euler  FilterMethod=Forward Euler  ControllerParametersSource=internal  P=0.0465149735787069  I=0.000103289667980039  UseKiTs=off  D=4.65424935363042  UseExternalDerivativeSource=off  N=43.499456893011  UseFilter=on  TunerSelectOption=Transfer Function Based (PID Tuner App)  InitialConditionSource=internal  InitialConditionForIntegrator=0  InitialConditionForFilter=0  DifferentiatorICPrevScaledInput=0  ExternalReset=none  TrackingMode=off  Kt=1  LimitOutput=off  SatLimitsSource=internal  UpperSaturationLimit=inf  LowerSaturationLimit=-inf  LinearizeAsGain=on  AntiWindupMode=none  Kb=1  LimitIntegrator=off  UpperIntegratorSaturationLimit=inf  LowerIntegratorSaturationLimit=-inf  POutMin=[]  POutMax=[]  IOutMin=[]  IOutMax=[]  DOutMin=[]  DOutMax=[]  NOutMin=[]  NOutMax=[]  SumOutMin=[]  SumOutMax=[]  SaturationOutMin=[]  SaturationOutMax=[]  PParamMin=[]  PParamMax=[]  IParamMin=[]  IParamMax=[]  DParamMin=[]  DParamMax=[]  NParamMin=[]  NParamMax=[]  KbParamMin=[]  KbParamMax=[]  KtParamMin=[]  KtParamMax=[]  KbOutMin=[]  KbOutMax=[]  KtOutMin=[]  KtOutMax=[]  IntegratorOutMin=[]  IntegratorOutMax=[]  FilterOutMin=[]  FilterOutMax=[]  SumI1OutMin=[]  SumI1OutMax=[]  SumI2OutMin=[]  SumI2OutMax=[]  SumI3OutMin=[]  SumI3OutMax=[]  SumI4OutMin=[]  SumI4OutMax=[]  SumDOutMin=[]  SumDOutMax=[]  DifferentiatorOutMin=[]  DifferentiatorOutMax=[]  FilterDiffOutCoefMin=[]  FilterDiffOutCoefMax=[]  ReciprocalOutMin=[]  ReciprocalOutMax=[]  SumDenOutMin=[]  SumDenOutMax=[]  SumNumOutMin=[]  SumNumOutMax=[]  DivideOutMin=[]  DivideOutMax=[]  UdiffTsProdOutMin=[]  UdiffTsProdOutMax=[]  NTsProdOutMin=[]  NTsProdOutMax=[]  UintegralTsProdOutMin=[]  UintegralTsProdOutMax=[]  UngainTsProdOutMin=[]  UngainTsProdOutMax=[]  ClampingZeroOutDataTypeStr=Inherit: Inherit via back propagation  ClampingZeroOutMin=[]  ClampingZeroOutMax=[]  FilterDenConstantOutDataTypeStr=Inherit: Inherit via back propagation  FilterDenConstantOutMin=[]  FilterDenConstantOutMax=[]  PCopyOutDataTypeStr=Inherit: Inherit via back propagation  PCopyOutMin=[]  PCopyOutMax=[]  NCopyOutDataTypeStr=Inherit: Inherit via back propagation  NCopyOutMin=[]  NCopyOutMax=[]  IntegratorContinuousStateAttributes=''  IntegratorStateMustResolveToSignalObject=off  IntegratorRTWStateStorageClass=Auto  FilterContinuousStateAttributes=''  FilterStateMustResolveToSignalObject=off  FilterRTWStateStorageClass=Auto  ParallelPVariant=InternalParameters  IdealPVariant=Disabled  IVariant=InternalParameters  DVariant=InternalParameters  IntegratorVariant=Continuous  SatVariant=Disabled  AWVariant=Passthrough  PCopyVariant=Disabled  TRVariant=Disabled  FdbkBlocksVariant=Forward  IdealPFdbkVariant=Disabled  SatFdbkVariant=Disabled  DerivativeFilterVariant=ContFilter  NVariant=InternalParameters  NCopyVariant=Disabled  FilterICVariant=InternalICsFilter  IntegratorICVariant=InternalICs  ExternalResetVariant=Disabled  TRSumVariant=Passthrough  SumFdbkVariant=Disabled  SumVariant=Sum_PID  TsampFilterVariant=InternalTs  TsampNgainVariant=Passthrough  TsampIntegralVariant=Disabled_SignalSpec  ExternalSaturationOutDataTypeStr=Inherit: Same as second input  DerivativeSourceVariant=ErrorSignal  PreIntVariant=InternalPreInt
  PID Controller1 : slpidlib/PID Controller  Commented=on  Controller=PID  Form=Parallel  TimeDomain=Continuous-time  UseExternalTs=off  SampleTime=-1  IntegratorMethod=Forward Euler  FilterMethod=Forward Euler  ControllerParametersSource=internal  P=-8.70356529470234  I=-0.000904169381532931  UseKiTs=off  D=-18615.1079342445  UseExternalDerivativeSource=off  N=2.03503712412566  UseFilter=on  TunerSelectOption=Transfer Function Based (PID Tuner App)  InitialConditionSource=internal  InitialConditionForIntegrator=0  InitialConditionForFilter=0  DifferentiatorICPrevScaledInput=0  ExternalReset=none  TrackingMode=off  Kt=1  LimitOutput=off  SatLimitsSource=internal  UpperSaturationLimit=inf  LowerSaturationLimit=-inf  LinearizeAsGain=on  AntiWindupMode=none  Kb=1  LimitIntegrator=off  UpperIntegratorSaturationLimit=inf  LowerIntegratorSaturationLimit=-inf  POutMin=[]  POutMax=[]  IOutMin=[]  IOutMax=[]  DOutMin=[]  DOutMax=[]  NOutMin=[]  NOutMax=[]  SumOutMin=[]  SumOutMax=[]  SaturationOutMin=[]  SaturationOutMax=[]  PParamMin=[]  PParamMax=[]  IParamMin=[]  IParamMax=[]  DParamMin=[]  DParamMax=[]  NParamMin=[]  NParamMax=[]  KbParamMin=[]  KbParamMax=[]  KtParamMin=[]  KtParamMax=[]  KbOutMin=[]  KbOutMax=[]  KtOutMin=[]  KtOutMax=[]  IntegratorOutMin=[]  IntegratorOutMax=[]  FilterOutMin=[]  FilterOutMax=[]  SumI1OutMin=[]  SumI1OutMax=[]  SumI2OutMin=[]  SumI2OutMax=[]  SumI3OutMin=[]  SumI3OutMax=[]  SumI4OutMin=[]  SumI4OutMax=[]  SumDOutMin=[]  SumDOutMax=[]  DifferentiatorOutMin=[]  DifferentiatorOutMax=[]  FilterDiffOutCoefMin=[]  FilterDiffOutCoefMax=[]  ReciprocalOutMin=[]  ReciprocalOutMax=[]  SumDenOutMin=[]  SumDenOutMax=[]  SumNumOutMin=[]  SumNumOutMax=[]  DivideOutMin=[]  DivideOutMax=[]  UdiffTsProdOutMin=[]  UdiffTsProdOutMax=[]  NTsProdOutMin=[]  NTsProdOutMax=[]  UintegralTsProdOutMin=[]  UintegralTsProdOutMax=[]  UngainTsProdOutMin=[]  UngainTsProdOutMax=[]  ClampingZeroOutDataTypeStr=Inherit: Inherit via back propagation  ClampingZeroOutMin=[]  ClampingZeroOutMax=[]  FilterDenConstantOutDataTypeStr=Inherit: Inherit via back propagation  FilterDenConstantOutMin=[]  FilterDenConstantOutMax=[]  PCopyOutDataTypeStr=Inherit: Inherit via back propagation  PCopyOutMin=[]  PCopyOutMax=[]  NCopyOutDataTypeStr=Inherit: Inherit via back propagation  NCopyOutMin=[]  NCopyOutMax=[]  IntegratorContinuousStateAttributes=''  IntegratorStateMustResolveToSignalObject=off  IntegratorRTWStateStorageClass=Auto  FilterContinuousStateAttributes=''  FilterStateMustResolveToSignalObject=off  FilterRTWStateStorageClass=Auto  ParallelPVariant=InternalParameters  IdealPVariant=Disabled  IVariant=InternalParameters  DVariant=InternalParameters  IntegratorVariant=Continuous  SatVariant=Disabled  AWVariant=Passthrough  PCopyVariant=Disabled  TRVariant=Disabled  FdbkBlocksVariant=Forward  IdealPFdbkVariant=Disabled  SatFdbkVariant=Disabled  DerivativeFilterVariant=ContFilter  NVariant=InternalParameters  NCopyVariant=Disabled  FilterICVariant=InternalICsFilter  IntegratorICVariant=InternalICs  ExternalResetVariant=Disabled  TRSumVariant=Passthrough  SumFdbkVariant=Disabled  SumVariant=Sum_PID  TsampFilterVariant=InternalTs  TsampNgainVariant=Passthrough  TsampIntegralVariant=Disabled_SignalSpec  ExternalSaturationOutDataTypeStr=Inherit: Same as second input  DerivativeSourceVariant=ErrorSignal  PreIntVariant=InternalPreInt
  PID Controller2 : slpidlib/PID Controller  Commented=on  Controller=PID  Form=Parallel  TimeDomain=Continuous-time  UseExternalTs=off  SampleTime=-1  IntegratorMethod=Forward Euler  FilterMethod=Forward Euler  ControllerParametersSource=internal  P=9.93439404723568  I=0.000287249258430092  UseKiTs=off  D=76338.7105026537  UseExternalDerivativeSource=off  N=0.566418286371796  UseFilter=on  TunerSelectOption=Transfer Function Based (PID Tuner App)  InitialConditionSource=internal  InitialConditionForIntegrator=0  InitialConditionForFilter=0  DifferentiatorICPrevScaledInput=0  ExternalReset=none  TrackingMode=off  Kt=1  LimitOutput=off  SatLimitsSource=internal  UpperSaturationLimit=inf  LowerSaturationLimit=-inf  LinearizeAsGain=on  AntiWindupMode=none  Kb=1  LimitIntegrator=off  UpperIntegratorSaturationLimit=inf  LowerIntegratorSaturationLimit=-inf  POutMin=[]  POutMax=[]  IOutMin=[]  IOutMax=[]  DOutMin=[]  DOutMax=[]  NOutMin=[]  NOutMax=[]  SumOutMin=[]  SumOutMax=[]  SaturationOutMin=[]  SaturationOutMax=[]  PParamMin=[]  PParamMax=[]  IParamMin=[]  IParamMax=[]  DParamMin=[]  DParamMax=[]  NParamMin=[]  NParamMax=[]  KbParamMin=[]  KbParamMax=[]  KtParamMin=[]  KtParamMax=[]  KbOutMin=[]  KbOutMax=[]  KtOutMin=[]  KtOutMax=[]  IntegratorOutMin=[]  IntegratorOutMax=[]  FilterOutMin=[]  FilterOutMax=[]  SumI1OutMin=[]  SumI1OutMax=[]  SumI2OutMin=[]  SumI2OutMax=[]  SumI3OutMin=[]  SumI3OutMax=[]  SumI4OutMin=[]  SumI4OutMax=[]  SumDOutMin=[]  SumDOutMax=[]  DifferentiatorOutMin=[]  DifferentiatorOutMax=[]  FilterDiffOutCoefMin=[]  FilterDiffOutCoefMax=[]  ReciprocalOutMin=[]  ReciprocalOutMax=[]  SumDenOutMin=[]  SumDenOutMax=[]  SumNumOutMin=[]  SumNumOutMax=[]  DivideOutMin=[]  DivideOutMax=[]  UdiffTsProdOutMin=[]  UdiffTsProdOutMax=[]  NTsProdOutMin=[]  NTsProdOutMax=[]  UintegralTsProdOutMin=[]  UintegralTsProdOutMax=[]  UngainTsProdOutMin=[]  UngainTsProdOutMax=[]  ClampingZeroOutDataTypeStr=Inherit: Inherit via back propagation  ClampingZeroOutMin=[]  ClampingZeroOutMax=[]  FilterDenConstantOutDataTypeStr=Inherit: Inherit via back propagation  FilterDenConstantOutMin=[]  FilterDenConstantOutMax=[]  PCopyOutDataTypeStr=Inherit: Inherit via back propagation  PCopyOutMin=[]  PCopyOutMax=[]  NCopyOutDataTypeStr=Inherit: Inherit via back propagation  NCopyOutMin=[]  NCopyOutMax=[]  IntegratorContinuousStateAttributes=''  IntegratorStateMustResolveToSignalObject=off  IntegratorRTWStateStorageClass=Auto  FilterContinuousStateAttributes=''  FilterStateMustResolveToSignalObject=off  FilterRTWStateStorageClass=Auto  ParallelPVariant=InternalParameters  IdealPVariant=Disabled  IVariant=InternalParameters  DVariant=InternalParameters  IntegratorVariant=Continuous  SatVariant=Disabled  AWVariant=Passthrough  PCopyVariant=Disabled  TRVariant=Disabled  FdbkBlocksVariant=Forward  IdealPFdbkVariant=Disabled  SatFdbkVariant=Disabled  DerivativeFilterVariant=ContFilter  NVariant=InternalParameters  NCopyVariant=Disabled  FilterICVariant=InternalICsFilter  IntegratorICVariant=InternalICs  ExternalResetVariant=Disabled  TRSumVariant=Passthrough  SumFdbkVariant=Disabled  SumVariant=Sum_PID  TsampFilterVariant=InternalTs  TsampNgainVariant=Passthrough  TsampIntegralVariant=Disabled_SignalSpec  ExternalSaturationOutDataTypeStr=Inherit: Same as second input  DerivativeSourceVariant=ErrorSignal  PreIntVariant=InternalPreInt
  Saturation : Saturate  UpperLimit=500  LowerLimit=-500
  Sum : Sum  Inputs=|+-
  Sum1 : Sum  Inputs=|+-
  Sum2 : Sum  Inputs=|+-
  Sum3 : Sum  Inputs=+++
  Sum4 : Sum  Commented=on  Inputs=+++
  Ux : Outport
  Uy : Outport  Port=2
  Uz : Outport  Port=3
  tag scope: G=global, xyz=global
  wires:
  yd/1 -> Sum1/1
  zd/1 -> Sum2/1
  zo/1 -> Sum2/2
  yo/1 -> Sum1/2
  xo/1 -> Sum/2
  xd/1 -> Sum/1
  Ki/1 -> Integrator/1
  Kd/1 -> Derivative/1
  Integrator/1 -> Sum3/2
  Kp/1 -> Sum3/1
  Derivative/1 -> Sum3/3
  PID Controller/1 -> Sum4/1
  PID Controller1/1 -> Sum4/2
  PID Controller2/1 -> Sum4/3
  Saturation/1 -> [G], Demux1/1
  Sum/1 -> Mux/1
  Sum1/1 -> Mux/2
  Sum2/1 -> Mux/3
  Demux1/1 -> Ux/1
  Demux1/2 -> Uy/1
  Demux1/3 -> Uz/1
  Mux/1 -> [xyz], Kd/1, Ki/1, Kp/1
  Sum3/1 -> Saturation/1

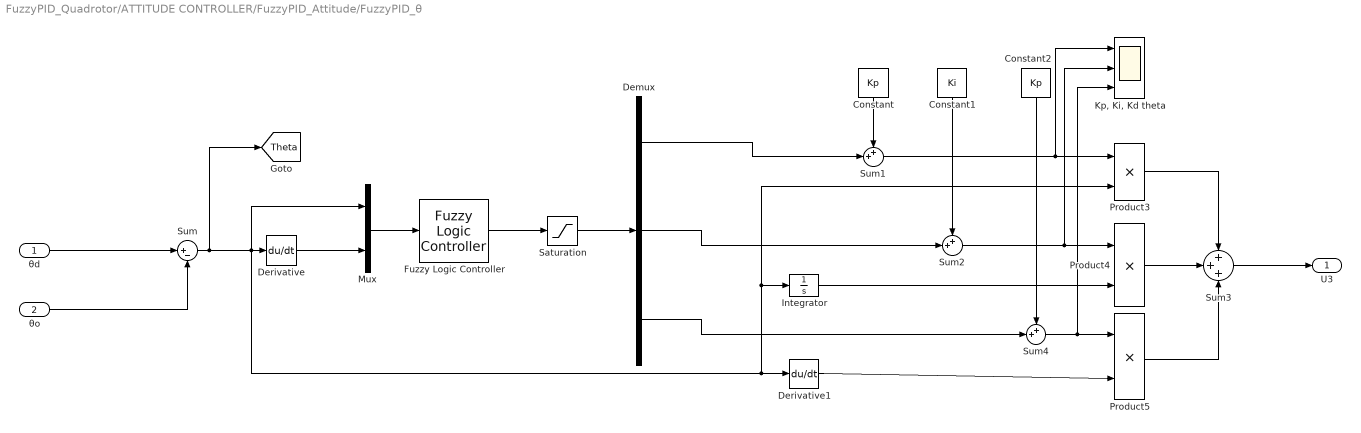
== system FuzzyPID_Quadrotor/ATTITUDE CONTROLLER/FuzzyPID_Attitude/FuzzyPID_θ ==
  θd : Inport
  θo : Inport  Port=2
  Constant : Constant  Value=Kp
  Constant1 : Constant  Value=Ki
  Constant2 : Constant  Value=Kp
  Demux : Demux  Outputs=3
  Derivative : Derivative
  Derivative1 : Derivative
  Fuzzy Logic Controller : fuzblock/Fuzzy Logic  Controller  FIS='FuzzyPID_Attitude.fis'  OutputSampleNumber=101  DataType=double  UseLookupTable=off  NumBreakpoints=10  FuzzifiedInputs=off  RuleFiringStrengths=off  RuleOutputs=off  AggregatedOutputs=off  SimulateUsing=Interpreted execution  OutOfRangeInputValueMessage=warning  NoRuleFiredMessage=warning  EmptyOutputFuzzySetMessage=warning
  Integrator : Integrator
  "Kp, Ki, Kd theta" : Scope  NumInputPorts=3
      settings: ActiveDisplayYMinimum=0.012410879904080067  ActiveDisplayYMaximum=62.956354195451212  DataLoggingVariableName=ScopeData7
  Mux : Mux  Inputs=2
  Product3 : Product
  Product4 : Product
  Product5 : Product
  Saturation : Saturate  UpperLimit=10  LowerLimit=-10
  Sum : Sum  Inputs=|+-
  Sum1 : Sum  Inputs=++|
  Sum2 : Sum  Inputs=++|
  Sum3 : Sum  Inputs=+++
  Sum4 : Sum  Inputs=++|
  U3 : Outport
  tag scope: Theta=global
  wires:
  Fuzzy Logic Controller/1 -> Saturation/1
  Constant/1 -> Sum1/1
  Derivative1/1 -> Product5/2
  Integrator/1 -> Product4/2
  Sum/1 -> [Theta], Mux/1, Product3/2, Integrator/1, Derivative1/1, Derivative/1
  Product4/1 -> Sum3/2
  Sum4/1 -> "Kp, Ki, Kd theta"/3, Product5/1
  Sum2/1 -> "Kp, Ki, Kd theta"/2, Product4/1
  Derivative/1 -> Mux/2
  Constant2/1 -> Sum4/1
  Constant1/1 -> Sum2/1
  Product3/1 -> Sum3/1
  Product5/1 -> Sum3/3
  Mux/1 -> Fuzzy Logic Controller/1
  Sum1/1 -> "Kp, Ki, Kd theta"/1, Product3/1
  Saturation/1 -> Demux/1
  θd/1 -> Sum/1
  θo/1 -> Sum/2
  Sum3/1 -> U3/1
  Demux/1 -> Sum1/2
  Demux/2 -> Sum2/2
  Demux/3 -> Sum4/2

== system FuzzyPID_Quadrotor/ATTITUDE CONTROLLER/FuzzyPID_Attitude/FuzzyPID_ψ ==
  ψd : Inport
  ψo : Inport  Port=2
  Constant : Constant  Value=Kp
  Constant1 : Constant  Value=Ki
  Constant2 : Constant  Value=Kp
  Demux : Demux  Outputs=3
  Derivative : Derivative
  Derivative1 : Derivative
  Fuzzy Logic Controller : fuzblock/Fuzzy Logic  Controller  FIS='FuzzyPID_Attitude.fis'  OutputSampleNumber=101  DataType=double  UseLookupTable=off  NumBreakpoints=10  FuzzifiedInputs=off  RuleFiringStrengths=off  RuleOutputs=off  AggregatedOutputs=off  SimulateUsing=Interpreted execution  OutOfRangeInputValueMessage=warning  NoRuleFiredMessage=warning  EmptyOutputFuzzySetMessage=warning
  Integrator : Integrator
  "Kp, Ki, Kd psi" : Scope  NumInputPorts=3
      settings: ActiveDisplayYMinimum=-9.0947304378612035  ActiveDisplayYMaximum=81.994983604570493  DataLoggingVariableName=ScopeData8
  Mux : Mux  Inputs=2
  Product3 : Product
  Product4 : Product
  Product5 : Product
  Saturation : Saturate  UpperLimit=10  LowerLimit=-10
  Sum : Sum  Inputs=|+-
  Sum1 : Sum  Inputs=++|
  Sum2 : Sum  Inputs=++|
  Sum3 : Sum  Inputs=+++
  Sum4 : Sum  Inputs=++|
  U4 : Outport
  tag scope: Psi=global
  wires:
  Fuzzy Logic Controller/1 -> Saturation/1
  Constant/1 -> Sum1/1
  Demux/1 -> Sum1/2
  Derivative1/1 -> Product5/2
  Integrator/1 -> Product4/2
  Sum/1 -> [Psi], Mux/1, Product3/2, Integrator/1, Derivative1/1, Derivative/1
  Product4/1 -> Sum3/2
  Sum4/1 -> "Kp, Ki, Kd psi"/3, Product5/1
  Sum2/1 -> "Kp, Ki, Kd psi"/2, Product4/1
  Derivative/1 -> Mux/2
  Constant2/1 -> Sum4/1
  Constant1/1 -> Sum2/1
  Product3/1 -> Sum3/1
  Product5/1 -> Sum3/3
  Mux/1 -> Fuzzy Logic Controller/1
  Demux/3 -> Sum4/2
  Sum1/1 -> "Kp, Ki, Kd psi"/1, Product3/1
  Saturation/1 -> Demux/1
  ψd/1 -> Sum/1
  ψo/1 -> Sum/2
  Sum3/1 -> U4/1
  Demux/2 -> Sum2/2

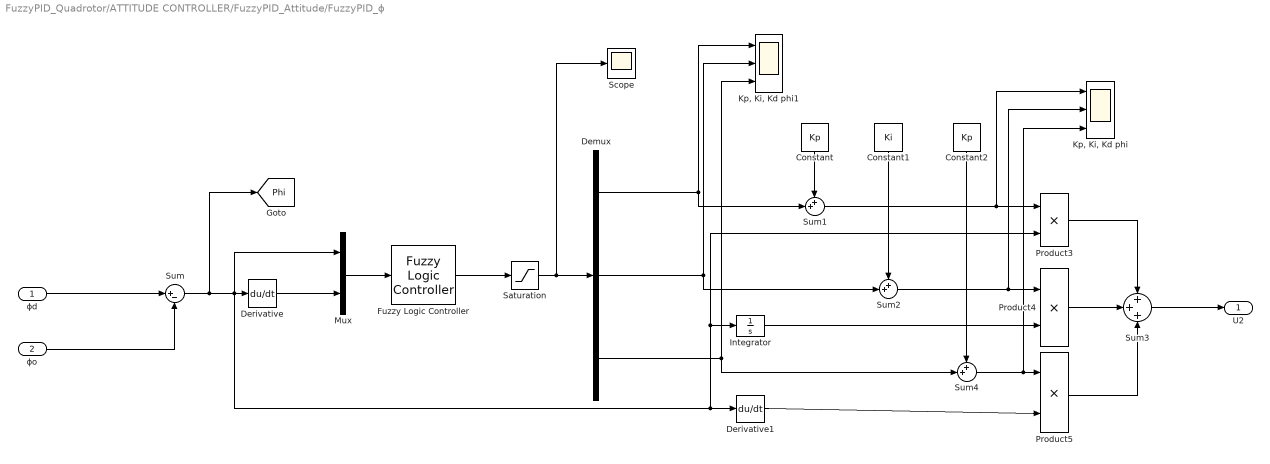
== system FuzzyPID_Quadrotor/ATTITUDE CONTROLLER/FuzzyPID_Attitude/FuzzyPID_ϕ ==
  ϕd : Inport
  ϕo : Inport  Port=2
  Constant : Constant  Value=Kp
  Constant1 : Constant  Value=Ki
  Constant2 : Constant  Value=Kp
  Demux : Demux  Outputs=3
  Derivative : Derivative
  Derivative1 : Derivative
  Fuzzy Logic Controller : fuzblock/Fuzzy Logic  Controller  FIS='FuzzyPID_Attitude.fis'  OutputSampleNumber=101  DataType=double  UseLookupTable=off  NumBreakpoints=10  FuzzifiedInputs=off  RuleFiringStrengths=off  RuleOutputs=off  AggregatedOutputs=off  SimulateUsing=Interpreted execution  OutOfRangeInputValueMessage=warning  NoRuleFiredMessage=warning  EmptyOutputFuzzySetMessage=warning
  Integrator : Integrator
  "Kp, Ki, Kd phi" : Scope  NumInputPorts=3
      settings: ActiveDisplayYMinimum=-1.0207579818789583  ActiveDisplayYMaximum=9.5994362022967916  DataLoggingVariableName=ScopeData6
  "Kp, Ki, Kd phi1" : Scope  NumInputPorts=3
      settings: ActiveDisplayYMinimum=-1.0634217305983689  ActiveDisplayYMaximum=10.104074379851752  DataLoggingVariableName=ScopeData10
  Mux : Mux  Inputs=2
  Product3 : Product
  Product4 : Product
  Product5 : Product
  Saturation : Saturate  UpperLimit=10  LowerLimit=-10
  Scope : Scope
      settings: ActiveDisplayYMinimum=-1.0634217305983689  ActiveDisplayYMaximum=10.104074379851752  DataLoggingVariableName=ScopeData9
  Sum : Sum  Inputs=|+-
  Sum1 : Sum  Inputs=++|
  Sum2 : Sum  Inputs=++|
  Sum3 : Sum  Inputs=+++
  Sum4 : Sum  Inputs=++|
  U2 : Outport
  tag scope: Phi=global
  wires:
  Demux/2 -> Sum2/2, "Kp, Ki, Kd phi1"/2
  Fuzzy Logic Controller/1 -> Saturation/1
  Constant/1 -> Sum1/1
  Demux/1 -> Sum1/2, "Kp, Ki, Kd phi1"/1
  Derivative1/1 -> Product5/2
  Integrator/1 -> Product4/2
  Sum/1 -> [Phi], Mux/1, Product3/2, Integrator/1, Derivative1/1, Derivative/1
  Product4/1 -> Sum3/2
  Sum4/1 -> "Kp, Ki, Kd phi"/3, Product5/1
  Sum2/1 -> "Kp, Ki, Kd phi"/2, Product4/1
  Derivative/1 -> Mux/2
  Constant2/1 -> Sum4/1
  Constant1/1 -> Sum2/1
  Product3/1 -> Sum3/1
  Product5/1 -> Sum3/3
  Mux/1 -> Fuzzy Logic Controller/1
  Demux/3 -> Sum4/2, "Kp, Ki, Kd phi1"/3
  Sum1/1 -> "Kp, Ki, Kd phi"/1, Product3/1
  Saturation/1 -> Scope/1, Demux/1
  ϕd/1 -> Sum/1
  ϕo/1 -> Sum/2
  Sum3/1 -> U2/1
